simulink subsystem "Linear_model"  (R2021b)
settings: Solver=VariableStepAuto  StartTime=0.0  StopTime=10.0  RelTol=1e-3
undefined symbols (not defined in the file): A, B, C, Q1, Q2
libraries: simulink x2
settings Model: Creator=aakas  LastModifiedBy=aakas

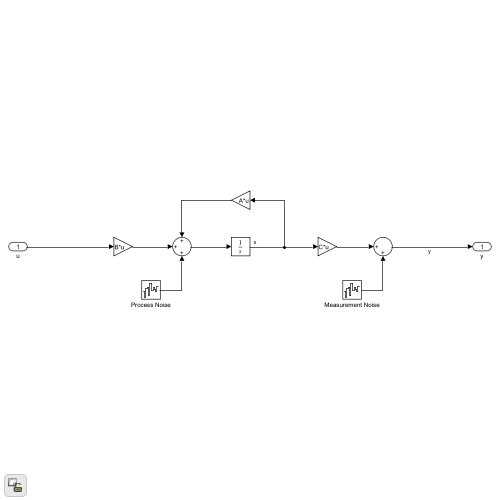
[thumbnail: Simulink's stored preview of the top-level diagram]
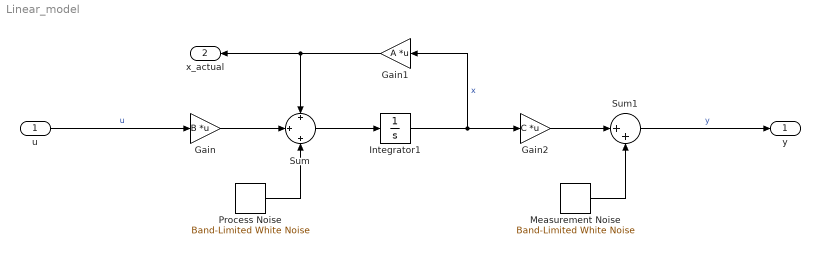
== system Linear_model ==
  u : Inport
  Gain : Gain  Gain=B  Multiplication=Matrix(K*u)
  Gain1 : Gain  Gain=A  Multiplication=Matrix(K*u)
  Gain2 : Gain  Gain=C  Multiplication=Matrix(K*u)
  Integrator1 : Integrator
  Measurement Noise : simulink/Sources/Band-Limited White Noise  Cov=R  Ts=0.1  seed=[32523]
  Process Noise : simulink/Sources/Band-Limited White Noise  Cov=[Q1; Q2]  Ts=0.1  seed=[23341]
  Sum : Sum  Inputs=+|+|+
  Sum1 : Sum  Inputs=|++
  y : Outport
  x_actual : Outport  Port=2
  wires:
  Integrator1/1 -> Gain1/1, Gain2/1  "x"
  u/1 -> Gain/1  "u"
  Gain2/1 -> Sum1/1
  Gain1/1 -> x_actual/1, Sum/1
  Gain/1 -> Sum/2
  Measurement Noise/1 -> Sum1/2
  Process Noise/1 -> Sum/3
  Sum/1 -> Integrator1/1
  Sum1/1 -> y/1  "y"
